simulink model "simulink_lab2_24b"  (R2024b)
settings: Solver=ode45  StartTime=0.0  StopTime=t_sim  MaxStep=0.0001*Ts  MinStep=0.00001*Ts  RelTol=1e-3
values from neighbouring files (symbols this model uses):
  d2 = 0    [LAB_PRACTICE_2_24b.m]
  rho = 3    [LAB_PRACTICE_2_24b.m]
  Ts = 0.01    [LAB_PRACTICE_2_24b.m]
libraries: cstblocks x2, simulink x1
settings Model: Creator=filoz  LastModifiedBy=filoz
settings SolverCC: InitialStep=0.00001*Ts

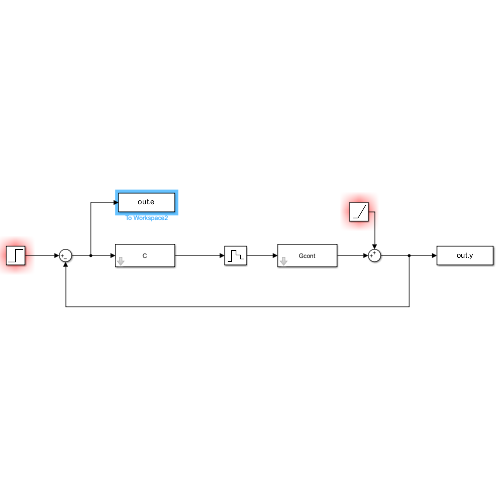
[thumbnail: Simulink's stored preview of the top-level diagram]
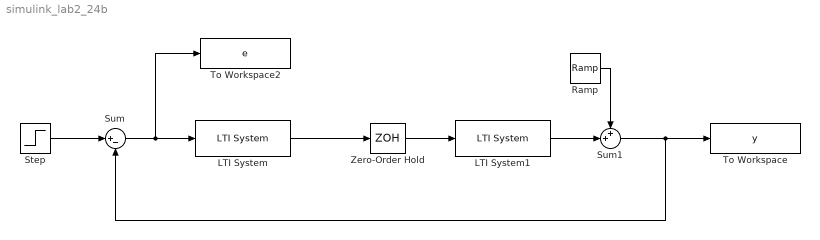
== system simulink_lab2_24b ==
  LTI System : cstblocks/LTI System  sys=C  IC=[]  PadeOrder=0
  LTI System1 : cstblocks/LTI System  sys=Gcont  IC=[]  PadeOrder=0
  Ramp : simulink/Sources/Ramp  slope=d2  start=0  InitialOutput=0
  Step : Step  Time=0  After=rho  SampleTime=Ts
  Sum : Sum  Inputs=|+-
  Sum1 : Sum  Inputs=++|
  To Workspace : ToWorkspace  VariableName=y  SaveFormat=Timeseries  SampleTime=Ts
  To Workspace2 : ToWorkspace  VariableName=e  SaveFormat=Timeseries  SampleTime=Ts
  Zero-Order Hold : ZeroOrderHold  SampleTime=Ts
  wires:
  Ramp/1 -> Sum1/1
  LTI System1/1 -> Sum1/2
  Sum1/1 -> Sum/2, To Workspace/1
  LTI System/1 -> Zero-Order Hold/1
  Zero-Order Hold/1 -> LTI System1/1
  Sum/1 -> To Workspace2/1, LTI System/1
  Step/1 -> Sum/1
